simulink model "SIR"  (R2017b)
settings: Solver=ode23  StartTime=0.0  StopTime=20  RelTol=1e-3
libraries: simulink x1
settings Model: Creator=jim  LastModifiedBy=jim

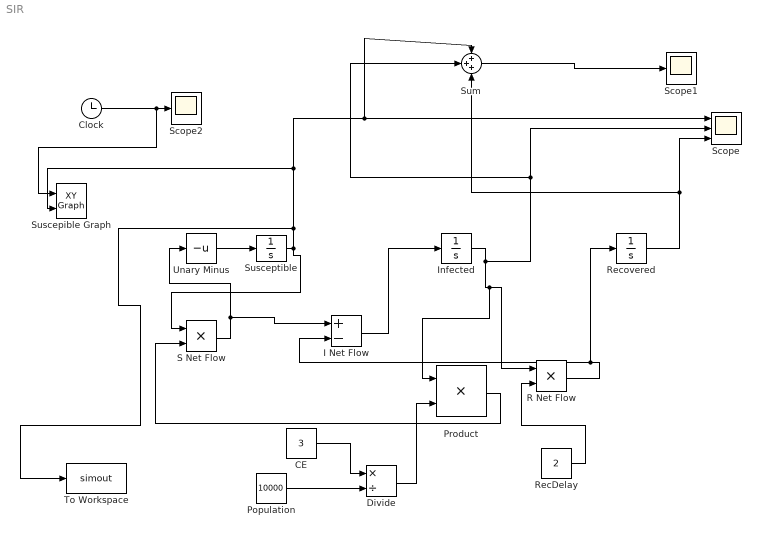
== system SIR ==
  CE : Constant  Value=3
  Clock : Clock
  Divide : Product  Inputs=*/
  I Net Flow : Sum  Inputs=+-
  Infected : Integrator  InitialCondition=1
  Population : Constant  Value=10000
  Product : Product
  R Net Flow : Product
  RecDelay : Constant  Value=2
  Recovered : Integrator
  S Net Flow : Product
  Scope : Scope  NumInputPorts=3
  Scope1 : Scope
  Scope2 : Scope
  Sum : Sum  Inputs=3
  Suscepible Graph : simulink/Sinks/XY Graph  xmin=0  xmax=20  ymin=0  ymax=10000  st=-1
  Susceptible : Integrator  InitialCondition=9999
  To Workspace : ToWorkspace  VariableName=simout  SaveFormat=Timeseries  SampleTime=-1
  Unary Minus : UnaryMinus
  wires:
  Infected/1 -> Sum/2, Scope/2, Product/1, R Net Flow/1
  Susceptible/1 -> Suscepible Graph/2, Sum/1, Scope/1, To Workspace/1, S Net Flow/1
  S Net Flow/1 -> I Net Flow/1, Unary Minus/1
  Unary Minus/1 -> Susceptible/1
  RecDelay/1 -> R Net Flow/2
  R Net Flow/1 -> Recovered/1, I Net Flow/2
  I Net Flow/1 -> Infected/1
  Recovered/1 -> Sum/3, Scope/3
  CE/1 -> Divide/1
  Population/1 -> Divide/2
  Divide/1 -> Product/2
  Product/1 -> S Net Flow/2
  Sum/1 -> Scope1/1
  Clock/1 -> Suscepible Graph/1, Scope2/1
